simulink model "Embedded_HW01_Q7"  (R2023a)
settings: Solver=VariableStepAuto  StartTime=0.0  StopTime=10.0  RelTol=1e-3
settings Model: Creator=reza  LastModifiedBy=reza

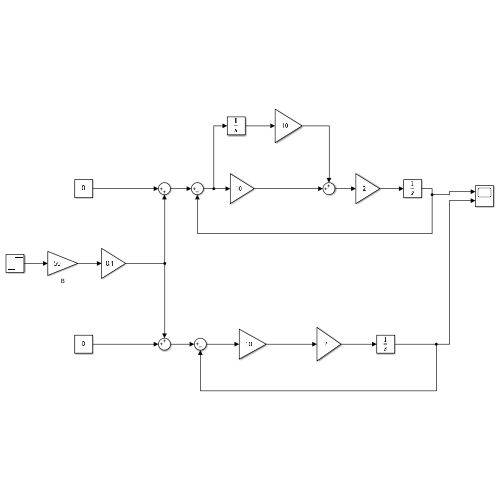
[thumbnail: Simulink's stored preview of the top-level diagram]
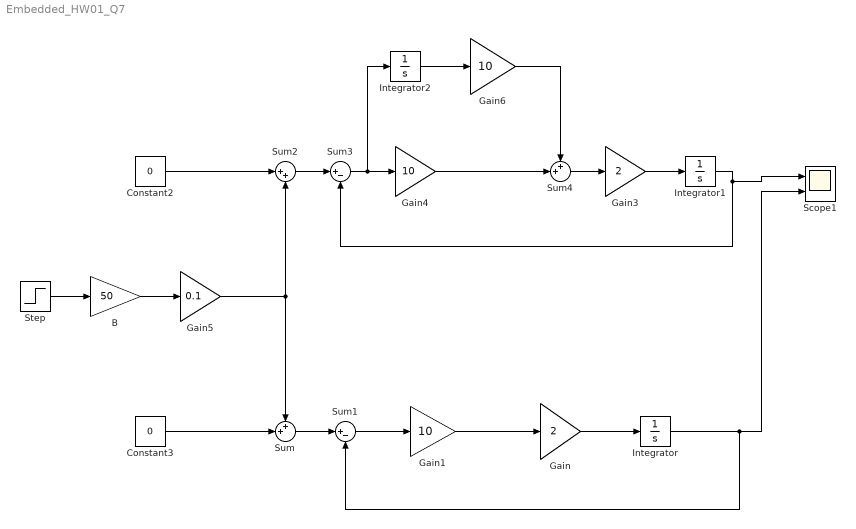
== system Embedded_HW01_Q7 ==
  B : Gain  Gain=50
  Constant2 : Constant  Value=0
  Constant3 : Constant  Value=0
  Gain : Gain  Gain=2
  Gain1 : Gain  Gain=10
  Gain3 : Gain  Gain=2
  Gain4 : Gain  Gain=10
  Gain5 : Gain  Gain=0.1
  Gain6 : Gain  Gain=10
  Integrator : Integrator
  Integrator1 : Integrator
  Integrator2 : Integrator
  Scope1 : Scope  NumInputPorts=2
  Step : Step  SampleTime=0
  Sum : Sum  Inputs=++|
  Sum1 : Sum  Inputs=|+-
  Sum2 : Sum  Inputs=|++
  Sum3 : Sum  Inputs=|+-
  Sum4 : Sum  Inputs=++|
  wires:
  Sum3/1 -> Integrator2/1, Gain4/1
  Integrator2/1 -> Gain6/1
  Gain5/1 -> Sum/1, Sum2/2
  Constant2/1 -> Sum2/1
  Gain6/1 -> Sum4/1
  Integrator1/1 -> Sum3/2, Scope1/1
  Constant3/1 -> Sum/2
  Gain4/1 -> Sum4/2
  Sum2/1 -> Sum3/1
  Gain1/1 -> Gain/1
  Sum4/1 -> Gain3/1
  Sum1/1 -> Gain1/1
  Gain/1 -> Integrator/1
  B/1 -> Gain5/1
  Sum/1 -> Sum1/1
  Step/1 -> B/1
  Gain3/1 -> Integrator1/1
  Integrator/1 -> Scope1/2, Sum1/2
